simulink model "chartTest"  (R2013b)
settings: Solver=ode45  StartTime=0.0  StopTime=30  RelTol=1e-3
settings Model: Creator=mainster  LastModifiedBy=mainster

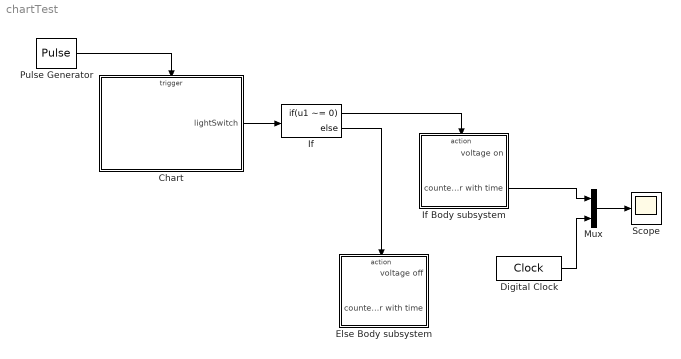
== system chartTest ==
  Chart : Stateflow chart  TreatAsAtomicUnit=on
  Digital Clock : DigitalClock
  Else Body subsystem : Subsystem  TreatAsAtomicUnit=on
  If : If  IfExpression=u1 ~= 0
  If Body subsystem : Subsystem  TreatAsAtomicUnit=on
  Mux : Mux  Inputs=2
  Pulse Generator : DiscretePulseGenerator  SampleTime=-1
  Scope : Scope
      settings: ShowLegends=on
  wires:
  Pulse Generator/1 -> Chart/Trigger
  Chart/1(lightSwitch) -> If/1
  If/1 -> If Body subsystem/Action
  If/2 -> Else Body subsystem/Action
  If Body subsystem/2(counter with time) -> Mux/1
  Digital Clock/1 -> Mux/2
  Mux/1 -> Scope/1

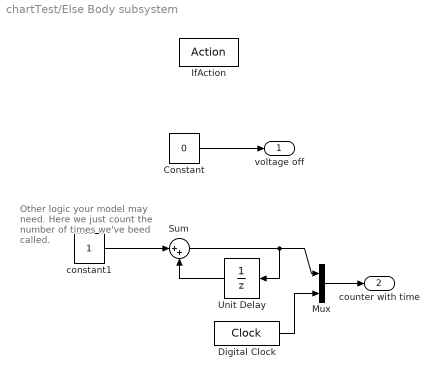
== system chartTest/Else Body subsystem ==
  note: Other logic your model may need. Here we just count the number
      | of times we've beed called.
  IfAction : ActionPort  ActionType=else
  Constant : Constant  Value=0
  Digital Clock : DigitalClock
  Mux : Mux  Inputs=2
  Sum : Sum  Inputs=|++  SaturateOnIntegerOverflow=on  InputSameDT=on  OutDataTypeStr=Inherit: Same as first input
  Unit Delay : UnitDelay
  constant1 : Constant
  voltage off : Outport  InitialOutput=0
  counter with time : Outport  Port=2
  wires:
  Constant/1 -> voltage off/1
  Sum/1 -> Mux/1, Unit Delay/1
  constant1/1 -> Sum/1
  Unit Delay/1 -> Sum/2
  Mux/1 -> counter with time/1
  Digital Clock/1 -> Mux/2

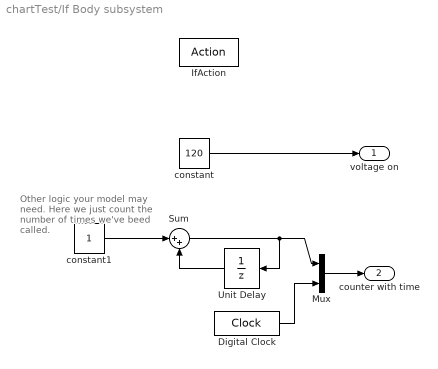
== system chartTest/If Body subsystem ==
  note: Other logic your model may need. Here we just count the number
      | of times we've beed called.
  IfAction : ActionPort  ActionType=then
  Digital Clock : DigitalClock
  Mux : Mux  Inputs=2
  Sum : Sum  Inputs=|++  SaturateOnIntegerOverflow=on  InputSameDT=on  OutDataTypeStr=Inherit: Same as first input
  Unit Delay : UnitDelay
  constant : Constant  Value=120
  constant1 : Constant
  voltage on : Outport  InitialOutput=120
  counter with time : Outport  Port=2
  wires:
  constant/1 -> voltage on/1
  Sum/1 -> Unit Delay/1, Mux/1
  constant1/1 -> Sum/1
  Unit Delay/1 -> Sum/2
  Mux/1 -> counter with time/1
  Digital Clock/1 -> Mux/2

== stateflow chart chartTest/Chart ==
  state on
  state off
  state ab
  on -> off [order 2] : switch/lightSwitch=0;
  on -> ab [order 1] : switch/lightSwitch=0.5;
  off -> ab : switch/lightSwitch=1;
  (default) -> off : /lightSwitch=0;
  data: lightSwitch output double
  events: switch input EITHER_EDGE_EVENT
